simulink model "Traffic_Light_StateFlow"  (R2018a)
settings: Solver=FixedStepDiscrete  StartTime=0.0  StopTime=10.0  RelTol=1e-3
settings Model: Creator=Moataz  LastModifiedBy=Moataz
settings OptimizationCC: DefaultParameterBehavior=Inlined  EnhancedBackFolding=on  PassReuseOutputArgsAs=Individual arguments  OptimizeBlockOrder=speed  DifferentSizesBufferReuse=on  OptimizationCustomize=off
settings DebuggingCC: ParameterTunabilityLossMsg=error
settings SFSimCC: MATLABDynamicMemAlloc=off
settings RTWCC: SystemTargetFile=ert.tlc  GenCodeOnly=on  TemplateMakefile=ert_default_tmf  GenerateReport=on  IncludeHyperlinkInReport=on  LaunchReport=on  GenerateTraceInfo=on  GenerateTraceReport=on  GenerateTraceReportSl=on  GenerateTraceReportSf=on  GenerateTraceReportEml=on
settings CodeAppCC: ForceParamTrailComments=on  IgnoreCustomStorageClasses=off  OperatorAnnotations=on  SimulinkDataObjDesc=on  SFDataObjDesc=on  InsertBlockDesc=on
settings ERTTargetCC: TargetLangStandard=C99 (ISO)  GenerateSampleERTMain=on  InlinedParameterPlacement=NonHierarchical  ERTCustomFileTemplate=example_file_process.tlc

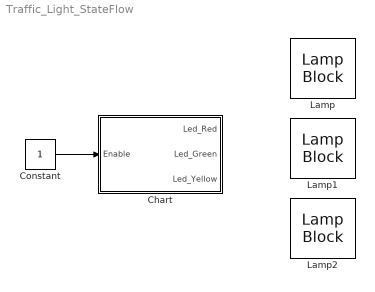
== system Traffic_Light_StateFlow ==
  Chart : Stateflow chart  TreatAsAtomicUnit=on
  Constant : Constant  OutDataTypeStr=boolean
  Lamp : LampBlock  WebBlockId=5
  Lamp1 : LampBlock  WebBlockId=8
  Lamp2 : LampBlock  WebBlockId=9
  wires:
  Constant/1 -> Chart/1(Enable)

== stateflow chart Traffic_Light_StateFlow/Chart ==
  state Traffic_Light
    state OFF
    state Red_ON
      en: %Enable RED_ON
      Led_Red=1;
      Counter=2;
      du:
      after(1,tick);
      Counter--;
      ex:
      Led_Red=0;
    state Yellow_ON
      en: %Enable Yellow_ON
      Led_Yellow=1;
      Counter=2;
      du:
      after(1,tick);
      Counter--;
      ex:
      Led_Yellow=0;
    state Green_ON
      en: %Enable Green_ON
      Led_Green=1;
      Counter=2;
      du:
      after(1,tick);
      Counter--;
      ex:
      Led_Green=0;
    (default) -> OFF
    OFF -> Red_ON : [Enable==1]
    Red_ON -> OFF [order 2] : [Enable==0]
    Green_ON -> Red_ON [order 1] : [Counter==0]
    Green_ON -> OFF [order 2] : [Enable==0]
    Yellow_ON -> OFF [order 2] : [Enable==0]
    Red_ON -> Yellow_ON [order 1] : [Counter==0]
    Yellow_ON -> Green_ON [order 1] : [Counter==0]
  (default) -> Traffic_Light
  data: Counter local uint8; Enable input boolean; EN local boolean; Led_Red output boolean; Led_Green output boolean; Led_Yellow output boolean
